simulink model "z5234550RundongGuanRun_DT1_2020"  (R2020a)
settings: Solver=ode4  StartTime=0.0  StopTime=1  FixedStep=1e-6  RelTol=1e-3
values from neighbouring files (symbols this model uses):
  FreqS = 52    [z5234550RundongGuanTestKiKp_DT1_2020.m]    (also in z5234550RundongGuanTestKi_DT1_2020.m; z5234550RundongGuanTestKp_DT1_2020.m)
  KI = ki(n)    [z5234550RundongGuanTestKiKp_DT1_2020.m]    (also in z5234550RundongGuanTestKi_DT1_2020.m; z5234550RundongGuanTestKp_DT1_2020.m = 100)
  KP = kp(m)    [z5234550RundongGuanTestKiKp_DT1_2020.m]    (also in z5234550RundongGuanTestKi_DT1_2020.m = 4; z5234550RundongGuanTestKp_DT1_2020.m = kp(n))
  m = 0.75    [z5234550RundongGuanTestKi_DT1_2020.m]    (also in z5234550RundongGuanTestKp_DT1_2020.m = 0.74)
  Tcs = 1e-4    (= 0.0001)    [z5234550RundongGuanInit_DT1_2020.m]    (also in z5234550RundongGuanSOGIBODE_DT1_2020.m; z5234550RundongGuanTestKiKp_DT1_2020.m; z5234550RundongGuanTestKi_DT1_2020.m; z5234550RundongGuanTestKp_DT1_2020.m)
undefined symbols (not defined in the file or in its folder): DiscIntNeverNeededParam
libraries: simulink x3
settings Model: SimulationMode=accelerator  Creator=slw  LastModifiedBy=Kevin
settings DataIOCC: ReturnWorkspaceOutputs=off
settings SFSimCC: CustomCodeUndefinedFunction=UseInterfaceOnly

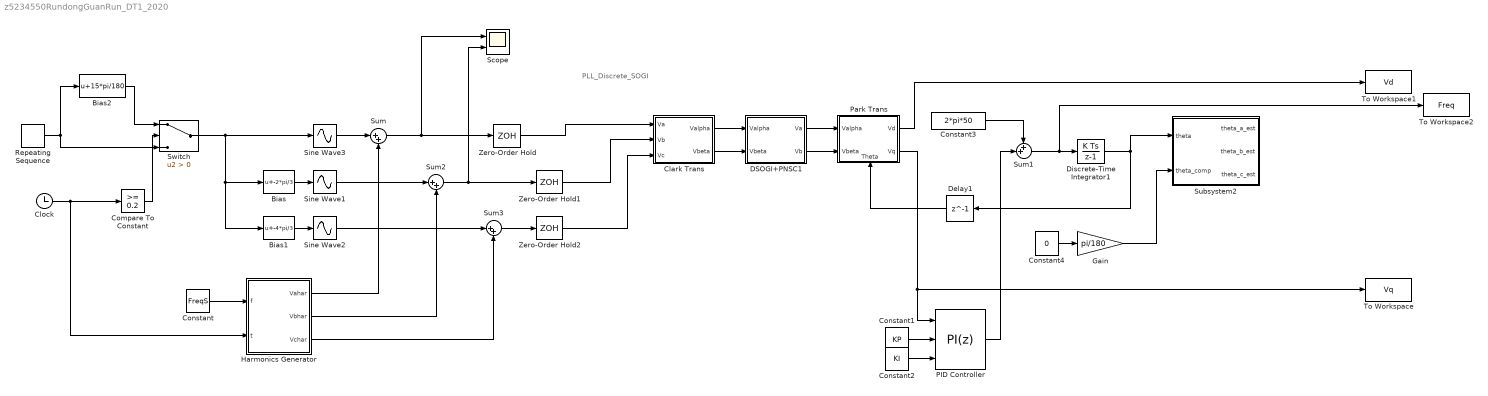
== system z5234550RundongGuanRun_DT1_2020 ==
  note: PLL_Discrete_SOGI
  Bias : Bias  Bias=-2*pi/3
  Bias1 : Bias  Bias=-4*pi/3
  Bias2 : Bias  Bias=15*pi/180
  Clark Trans : Subsystem
  Clock : Clock
  Compare To Constant : simulink/Logic and Bit Operations/Compare To Constant  relop=>=  const=0.2  OutDataTypeStr=boolean
  Constant : Constant  Value=FreqS
  Constant1 : Constant  Value=KP
  Constant2 : Constant  Value=KI
  Constant3 : Constant  Value=2*pi*50  SampleTime=Tcs
  Constant4 : Constant  Value=0
  DSOGI+PNSC1 : Subsystem
  Delay1 : Delay  DelayLength=1  SampleTime=Tcs
  Discrete-Time Integrator1 : DiscreteIntegrator  SampleTime=Tcs  ICPrevOutput=DiscIntNeverNeededParam  ICPrevScaledInput=DiscIntNeverNeededParam
  Gain : Gain  Gain=pi/180
  Harmonics Generator : MATLAB Function  TreatAsAtomicUnit=on
  PID Controller : simulink/Continuous/PID Controller  Controller=PI  Form=Parallel  TimeDomain=Discrete-time  UseExternalTs=off  SampleTime=1/10e3  IntegratorMethod=Forward Euler  FilterMethod=Forward Euler  ControllerParametersSource=external  P=20  I=0  D=0  UseFilter=on  N=100  TunerSelectOption=Transfer Function Based (PID Tuner App)  InitialConditionSource=internal  InitialConditionForIntegrator=0  InitialConditionForFilter=0  DifferentiatorICPrevScaledInput=0  ExternalReset=none  TrackingMode=off  Kt=1  LimitOutput=off  UpperSaturationLimit=inf  LowerSaturationLimit=-inf  LinearizeAsGain=on  AntiWindupMode=none  Kb=1  POutMin=[]  POutMax=[]  IOutMin=[]  IOutMax=[]  DOutMin=[]  DOutMax=[]  NOutMin=[]  NOutMax=[]  SumOutMin=[]  SumOutMax=[]  SaturationOutMin=[]  SaturationOutMax=[]  PParamMin=[]  PParamMax=[]  IParamMin=[]  IParamMax=[]  DParamMin=[]  DParamMax=[]  NParamMin=[]  NParamMax=[]  KbParamMin=[]  KbParamMax=[]  KtParamMin=[]  KtParamMax=[]  KbOutMin=[]  KbOutMax=[]  KtOutMin=[]  KtOutMax=[]  IntegratorOutMin=[]  IntegratorOutMax=[]  FilterOutMin=[]  FilterOutMax=[]  SumI1OutMin=[]  SumI1OutMax=[]  SumI2OutMin=[]  SumI2OutMax=[]  SumI3OutMin=[]  SumI3OutMax=[]  SumI4OutMin=[]  SumI4OutMax=[]  SumDOutMin=[]  SumDOutMax=[]  DifferentiatorOutMin=[]  DifferentiatorOutMax=[]  FilterDiffOutCoefMin=[]  FilterDiffOutCoefMax=[]  ReciprocalOutMin=[]  ReciprocalOutMax=[]  SumDenOutMin=[]  SumDenOutMax=[]  SumNumOutMin=[]  SumNumOutMax=[]  DivideOutMin=[]  DivideOutMax=[]  UdiffTsProdOutMin=[]  UdiffTsProdOutMax=[]  NTsProdOutMin=[]  NTsProdOutMax=[]  UintegralTsProdOutMin=[]  UintegralTsProdOutMax=[]  UngainTsProdOutMin=[]  UngainTsProdOutMax=[]  IntegratorContinuousStateAttributes=''  IntegratorStateMustResolveToSignalObject=off  IntegratorRTWStateStorageClass=Auto  FilterContinuousStateAttributes=''  FilterStateMustResolveToSignalObject=off  FilterRTWStateStorageClass=Auto  ParallelPVariant=ExternalParameters  IdealPVariant=Disabled  IVariant=ExternalParameters  DVariant=Disabled  IntegratorVariant=Discrete  SatVariant=Disabled  AWVariant=Passthrough  PCopyVariant=Disabled  TRVariant=Disabled  FdbkBlocksVariant=Forward  IdealPFdbkVariant=Disabled  SatFdbkVariant=Disabled  DerivativeFilterVariant=Disabled  NVariant=Disabled  NCopyVariant=Disabled_SignalSpec  FilterICVariant=Disabled  IntegratorICVariant=InternalICs  ExternalResetVariant=Disabled  TRSumVariant=Passthrough  SumFdbkVariant=Disabled  SumVariant=Sum_PI  TsampFilterVariant=InternalTs  TsampNgainVariant=Passthrough  TsampIntegralVariant=Passthrough
  Park Trans : Subsystem
      settings: PortSchema="{\"entries\":[{\"content\":{\"sides\":[{\"content\":{\"connectorIds\":[\"In1\",\"In2\"]},\"type\":\"ConnectorPlacement.EquallySpacedRectSide\",\"uuid\":\"d7ee73cc-3741-4077-b32c-689f2c701f83\"},{\"content\":{\"connectorIds\":[\"Out1\",\"Out2\"],\"side\":\"RIGHT\"},\"type\":\"ConnectorPlacement.EquallySpacedRectSide\",\"uuid\":\"fa84044a-ecd8-49d8-a4b2-ae549d89fe8f\"},{\"content\":{\"connectorIds\":[],\"side\":\"TOP\"},\"type\":\"ConnectorPlacement.EquallySpacedRectSide\",\"uuid\":\"692e7773-1833-4597-a5fd-7846ecf4550e\"},{\"content\":{\"connectorIds\":[\"In3\"],\"side\":\"BOTTOM\"},\"type\":\"ConnectorPlacement.EquallySpacedRectSide\",\"uuid\":\"73d654b9-9f56-4244-9824-eb13bf44a38f\"}]},\"type\":\"ConnectorPlacement.EquallySpacedConnector\",\"uuid\":\"4e0b4972-389e-416e-b0d9-9fdc8ba0f1f7\"}],\"packageUris\":[\"http://schema.mathworks.com/mf0/Connector/19700101\"],\"version\":\"1.0\"}"
  Repeating Sequence : simulink/Sources/Repeating Sequence  rep_seq_t=[0 1/FreqS]  rep_seq_y=[0 2*pi]
  Scope : Scope  NumInputPorts=2
  Sine Wave1 : Sin  TimeSource=Use external signal  Amplitude=230*sqrt(2)  SampleTime=0
  Sine Wave2 : Sin  TimeSource=Use external signal  Amplitude=230*sqrt(2)  SampleTime=0
  Sine Wave3 : Sin  TimeSource=Use external signal  Amplitude=230*sqrt(2)  SampleTime=0
  Subsystem2 : Subsystem
  Sum : Sum  Inputs=|++
  Sum1 : Sum  Inputs=++|
  Sum2 : Sum  Inputs=|++
  Sum3 : Sum  Inputs=|++
  Switch : Switch  Criteria=u2 > Threshold
  To Workspace : ToWorkspace  VariableName=Vq  SampleTime=-1
      settings: Save2DSignal=2-D array (concatenate along first dimension)
  To Workspace1 : ToWorkspace  VariableName=Vd  SampleTime=-1
      settings: Save2DSignal=2-D array (concatenate along first dimension)
  To Workspace2 : ToWorkspace  VariableName=Freq  SampleTime=-1
      settings: Save2DSignal=2-D array (concatenate along first dimension)
  Zero-Order Hold : ZeroOrderHold  SampleTime=Tcs
  Zero-Order Hold1 : ZeroOrderHold  SampleTime=Tcs
  Zero-Order Hold2 : ZeroOrderHold  SampleTime=Tcs
  wires:
  Repeating Sequence/1 -> Switch/3, Bias2/1
  Bias/1 -> Sine Wave1/1
  Bias1/1 -> Sine Wave2/1
  Switch/1 -> Bias1/1, Bias/1, Sine Wave3/1
  Bias2/1 -> Switch/1
  Clock/1 -> Harmonics Generator/2(t), Compare To Constant/1
  Compare To Constant/1 -> Switch/2
  Constant1/1 -> PID Controller/2
  Constant2/1 -> PID Controller/3
  Sum1/1 -> To Workspace2/1, Discrete-Time Integrator1/1
  Park Trans/2(Vq) -> To Workspace/1, PID Controller/1
  Clark Trans/1(Valpha) -> DSOGI+PNSC1/1(Valpha)
  Clark Trans/2(Vbeta) -> DSOGI+PNSC1/2(Vbeta)
  DSOGI+PNSC1/1(Va) -> Park Trans/1(Valpha)
  DSOGI+PNSC1/2(Vb) -> Park Trans/2(Vbeta)
  Delay1/1 -> Park Trans/3(Theta)
  Constant3/1 -> Sum1/1
  Discrete-Time Integrator1/1 -> Delay1/1, Subsystem2/1(theta)
  Park Trans/1(Vd) -> To Workspace1/1
  Constant4/1 -> Gain/1
  Gain/1 -> Subsystem2/2(theta_comp)
  PID Controller/1 -> Sum1/2
  Constant/1 -> Harmonics Generator/1(f)
  Sine Wave3/1 -> Sum/1
  Sum/1 -> Scope/1, Zero-Order Hold/1
  Sine Wave2/1 -> Sum3/1
  Sine Wave1/1 -> Sum2/1
  Sum2/1 -> Scope/2, Zero-Order Hold1/1
  Sum3/1 -> Zero-Order Hold2/1
  Harmonics Generator/1(Vahar) -> Sum/2
  Harmonics Generator/2(Vbhar) -> Sum2/2
  Harmonics Generator/3(Vchar) -> Sum3/2
  Zero-Order Hold/1 -> Clark Trans/1(Va)
  Zero-Order Hold1/1 -> Clark Trans/2(Vb)
  Zero-Order Hold2/1 -> Clark Trans/3(Vc)

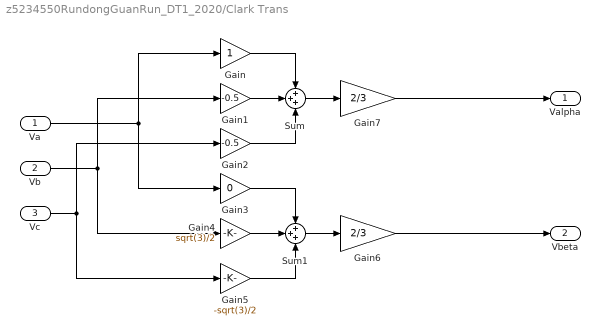
== system z5234550RundongGuanRun_DT1_2020/Clark Trans ==
  Va : Inport
  Vb : Inport  Port=2
  Vc : Inport  Port=3
  Gain : Gain
  Gain1 : Gain  Gain=-0.5
  Gain2 : Gain  Gain=-0.5
  Gain3 : Gain  Gain=0
  Gain4 : Gain  Gain=sqrt(3)/2
  Gain5 : Gain  Gain=-sqrt(3)/2
  Gain6 : Gain  Gain=2/3
  Gain7 : Gain  Gain=2/3
  Sum : Sum  Inputs=+++
  Sum1 : Sum  Inputs=+++
  Valpha : Outport
  Vbeta : Outport  Port=2
  wires:
  Gain6/1 -> Vbeta/1
  Gain7/1 -> Valpha/1
  Sum1/1 -> Gain6/1
  Sum/1 -> Gain7/1
  Gain4/1 -> Sum1/2
  Gain5/1 -> Sum1/3
  Gain1/1 -> Sum/2
  Gain3/1 -> Sum1/1
  Gain/1 -> Sum/1
  Vb/1 -> Gain1/1, Gain4/1
  Vc/1 -> Gain2/1, Gain5/1
  Va/1 -> Gain/1, Gain3/1
  Gain2/1 -> Sum/3

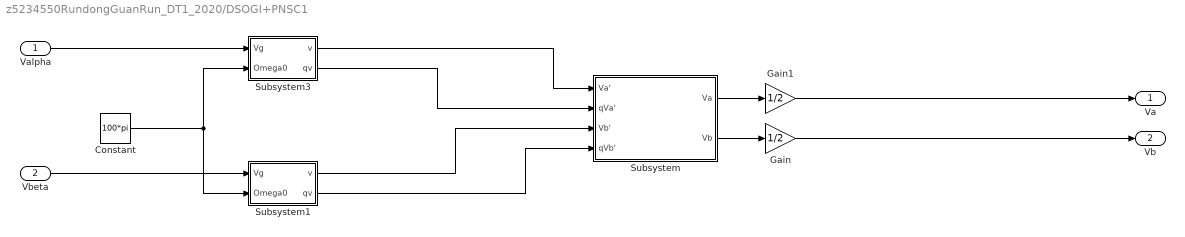
== system z5234550RundongGuanRun_DT1_2020/DSOGI+PNSC1 ==
  Valpha : Inport
  Vbeta : Inport  Port=2
  Constant : Constant  Value=100*pi
  Gain : Gain  Gain=1/2
  Gain1 : Gain  Gain=1/2
  Subsystem : Subsystem
  Subsystem1 : Subsystem
  Subsystem3 : Subsystem
  Va : Outport
  Vb : Outport  Port=2
  wires:
  Gain/1 -> Vb/1
  Gain1/1 -> Va/1
  Subsystem1/2(qv) -> Subsystem/4(qVb')
  Subsystem1/1(v) -> Subsystem/3(Vb')
  Vbeta/1 -> Subsystem1/1(Vg)
  Valpha/1 -> Subsystem3/1(Vg)
  Subsystem/2(Vb) -> Gain/1
  Subsystem/1(Va) -> Gain1/1
  Subsystem3/2(qv) -> Subsystem/2(qVa')
  Subsystem3/1(v) -> Subsystem/1(Va')
  Constant/1 -> Subsystem3/2(Omega0), Subsystem1/2(Omega0)

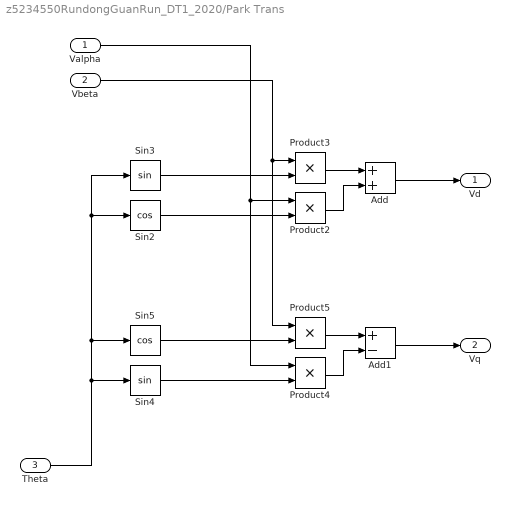
== system z5234550RundongGuanRun_DT1_2020/Park Trans ==
  Valpha : Inport
  Vbeta : Inport  Port=2
  Theta : Inport  Port=3
  Add : Sum
  Add1 : Sum  Inputs=+-
  Product{2..5} (4 alike) : Product
  Sin2 : Trigonometry  Operator=cos
  Sin3 : Trigonometry
  Sin4 : Trigonometry
  Sin5 : Trigonometry  Operator=cos
  Vd : Outport
  Vq : Outport  Port=2
  wires:
  Product5/1 -> Add1/1
  Sin4/1 -> Product4/2
  Add1/1 -> Vq/1
  Product3/1 -> Add/1
  Sin3/1 -> Product3/2
  Add/1 -> Vd/1
  Sin2/1 -> Product2/2
  Product2/1 -> Add/2
  Product4/1 -> Add1/2
  Valpha/1 -> Product4/1, Product2/1
  Sin5/1 -> Product5/2
  Theta/1 -> Sin3/1, Sin2/1, Sin5/1, Sin4/1
  Vbeta/1 -> Product3/1, Product5/1

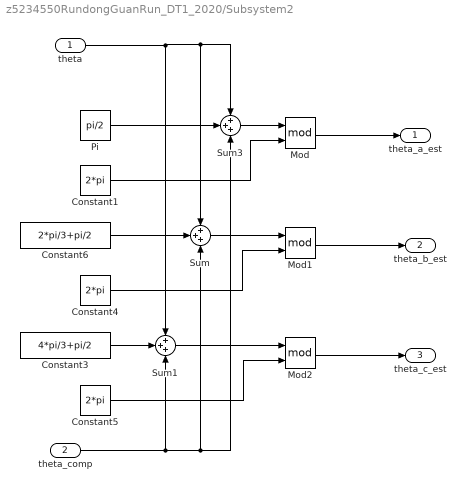
== system z5234550RundongGuanRun_DT1_2020/Subsystem2 ==
  theta : Inport
  theta_comp : Inport  Port=2
  Constant1 : Constant  Value=2*pi
  Constant3 : Constant  Value=4*pi/3+pi/2
  Constant4 : Constant  Value=2*pi
  Constant5 : Constant  Value=2*pi
  Constant6 : Constant  Value=2*pi/3+pi/2
  Mod : Math  Operator=mod  SaturateOnIntegerOverflow=on
  Mod1 : Math  Operator=mod  SaturateOnIntegerOverflow=on
  Mod2 : Math  Operator=mod  SaturateOnIntegerOverflow=on
  Pi : Constant  Value=pi/2  OutDataTypeStr=Inherit: Inherit via back propagation
  Sum : Sum  Inputs=+++
  Sum1 : Sum  Inputs=+++
  Sum3 : Sum  Inputs=+++
  theta_a_est : Outport
  theta_b_est : Outport  Port=2
  theta_c_est : Outport  Port=3
  wires:
  theta_comp/1 -> Sum3/3, Sum/3, Sum1/3
  Pi/1 -> Sum3/2
  Constant1/1 -> Mod/2
  Constant5/1 -> Mod2/2
  Sum/1 -> Mod1/1
  Sum3/1 -> Mod/1
  Constant3/1 -> Sum1/2
  Constant6/1 -> Sum/2
  Mod/1 -> theta_a_est/1
  theta/1 -> Sum/1, Sum3/1, Sum1/1
  Constant4/1 -> Mod1/2
  Sum1/1 -> Mod2/1
  Mod1/1 -> theta_b_est/1
  Mod2/1 -> theta_c_est/1

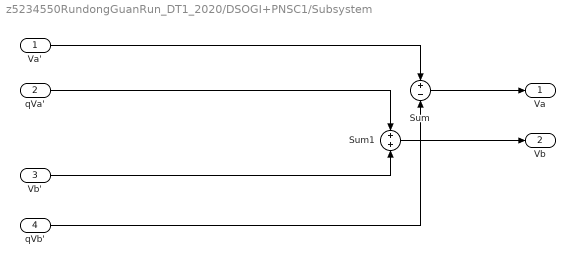
== system z5234550RundongGuanRun_DT1_2020/DSOGI+PNSC1/Subsystem ==
  Va' : Inport
  qVa' : Inport  Port=2
  Vb' : Inport  Port=3
  qVb' : Inport  Port=4
  Sum : Sum  Inputs=+|-
  Sum1 : Sum  Inputs=+|+
  Va : Outport
  Vb : Outport  Port=2
  wires:
  qVb'/1 -> Sum/2
  qVa'/1 -> Sum1/1
  Vb'/1 -> Sum1/2
  Va'/1 -> Sum/1
  Sum/1 -> Va/1
  Sum1/1 -> Vb/1

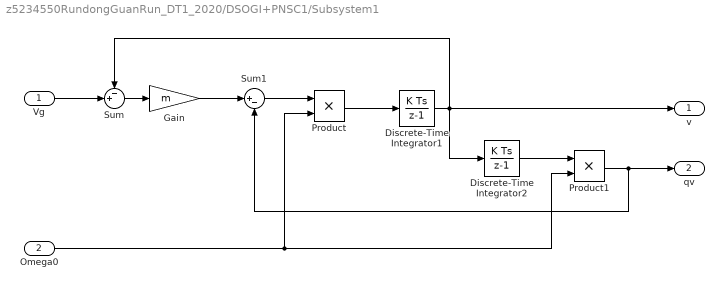
== system z5234550RundongGuanRun_DT1_2020/DSOGI+PNSC1/Subsystem1 ==
  Vg : Inport
  Omega0 : Inport  Port=2
  Discrete-Time Integrator1 : DiscreteIntegrator  gainval=1  SampleTime=Tcs  ICPrevOutput=DiscIntNeverNeededParam  ICPrevScaledInput=DiscIntNeverNeededParam
  Discrete-Time Integrator2 : DiscreteIntegrator  gainval=1  SampleTime=Tcs  ICPrevOutput=DiscIntNeverNeededParam  ICPrevScaledInput=DiscIntNeverNeededParam
  Gain : Gain  Gain=m
  Product : Product
  Product1 : Product
  Sum : Sum  Inputs=-+|
  Sum1 : Sum  Inputs=|+-
  v : Outport
  qv : Outport  Port=2
  wires:
  Sum/1 -> Gain/1
  Discrete-Time Integrator1/1 -> v/1, Sum/1, Discrete-Time Integrator2/1
  Omega0/1 -> Product1/2, Product/2
  Product/1 -> Discrete-Time Integrator1/1
  Discrete-Time Integrator2/1 -> Product1/1
  Product1/1 -> qv/1, Sum1/2
  Vg/1 -> Sum/2
  Gain/1 -> Sum1/1
  Sum1/1 -> Product/1

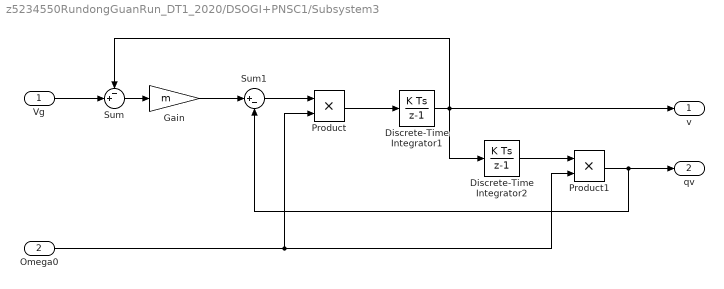
== system z5234550RundongGuanRun_DT1_2020/DSOGI+PNSC1/Subsystem3 ==
  Vg : Inport
  Omega0 : Inport  Port=2
  Discrete-Time Integrator1 : DiscreteIntegrator  gainval=1  SampleTime=Tcs  ICPrevOutput=DiscIntNeverNeededParam  ICPrevScaledInput=DiscIntNeverNeededParam
  Discrete-Time Integrator2 : DiscreteIntegrator  gainval=1  SampleTime=Tcs  ICPrevOutput=DiscIntNeverNeededParam  ICPrevScaledInput=DiscIntNeverNeededParam
  Gain : Gain  Gain=m
  Product : Product
  Product1 : Product
  Sum : Sum  Inputs=-+|
  Sum1 : Sum  Inputs=|+-
  v : Outport
  qv : Outport  Port=2
  wires:
  Sum1/1 -> Product/1
  Gain/1 -> Sum1/1
  Vg/1 -> Sum/2
  Product1/1 -> Sum1/2, qv/1
  Discrete-Time Integrator2/1 -> Product1/1
  Product/1 -> Discrete-Time Integrator1/1
  Omega0/1 -> Product/2, Product1/2
  Discrete-Time Integrator1/1 -> Discrete-Time Integrator2/1, Sum/1, v/1
  Sum/1 -> Gain/1

== matlab function z5234550RundongGuanRun_DT1_2020/Harmonics Generator ==
  data: f input; Vahar output; t input; Vbhar output; Vchar output
function [Vahar, Vbhar, Vchar] = fcn(f,t)
k=[3; 5; 7; 9; 11; 13];
Vk=[0.51;2.08;3.00;0.28;0.55;0.61];
ps=[101.4; 223.8; 121.3; -70.4; 201.4; 53.1];
Vahar=0;
Vbhar=0;
Vchar=0;

for i = 1:6
    Vahar = Vahar+Vk(i)*sin(k(i)*(2*pi*f*t)+ps(i));
    Vbhar = Vbhar+Vk(i)*sin(k(i)*(2*pi*f*t-2*pi/3)+ps(i));
    Vchar = Vchar+Vk(i)*sin(k(i)*(2*pi*f*t-4*pi/3)+ps(i));
end
